simulink model "TST_ActMod_TrqCalc"  (R2016b)
settings: Solver=FixedStepDiscrete  StartTime=0.0  StopTime=0.04  FixedStep=sampleTime  RelTol=1e-3
values from neighbouring files (symbols this model uses):
  testCase = 1    [initTST_ActMod_TrqCalc_001.m]
libraries: simulink x7, UnitTest_Lib x5
settings Model: Creator=caijinkang  LastModifiedBy=caijinkang
settings DebuggingCC: SignalRangeChecking=error

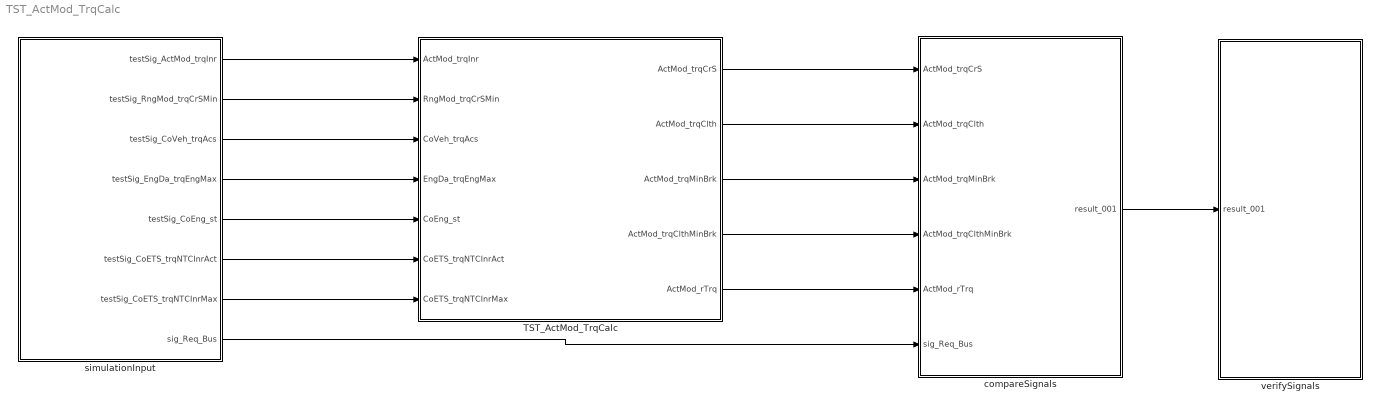
== system TST_ActMod_TrqCalc ==
  TST_ActMod_TrqCalc : Subsystem
  compareSignals : Subsystem
  simulationInput : Subsystem
  verifySignals : Subsystem
  wires:
  simulationInput/1(testSig_ActMod_trqInr) -> TST_ActMod_TrqCalc/1(ActMod_trqInr)
  simulationInput/2(testSig_RngMod_trqCrSMin) -> TST_ActMod_TrqCalc/2(RngMod_trqCrSMin)
  simulationInput/3(testSig_CoVeh_trqAcs) -> TST_ActMod_TrqCalc/3(CoVeh_trqAcs)
  simulationInput/4(testSig_EngDa_trqEngMax) -> TST_ActMod_TrqCalc/4(EngDa_trqEngMax)
  simulationInput/5(testSig_CoEng_st) -> TST_ActMod_TrqCalc/5(CoEng_st)
  simulationInput/6(testSig_CoETS_trqNTCInrAct) -> TST_ActMod_TrqCalc/6(CoETS_trqNTCInrAct)
  simulationInput/7(testSig_CoETS_trqNTCInrMax) -> TST_ActMod_TrqCalc/7(CoETS_trqNTCInrMax)
  TST_ActMod_TrqCalc/1(ActMod_trqCrS) -> compareSignals/1(ActMod_trqCrS)
  TST_ActMod_TrqCalc/2(ActMod_trqClth) -> compareSignals/2(ActMod_trqClth)
  TST_ActMod_TrqCalc/3(ActMod_trqMinBrk) -> compareSignals/3(ActMod_trqMinBrk)
  TST_ActMod_TrqCalc/4(ActMod_trqClthMinBrk) -> compareSignals/4(ActMod_trqClthMinBrk)
  TST_ActMod_TrqCalc/5(ActMod_rTrq) -> compareSignals/5(ActMod_rTrq)
  simulationInput/8(sig_Req_Bus) -> compareSignals/6(sig_Req_Bus)
  compareSignals/1(result_001) -> verifySignals/1(result_001)

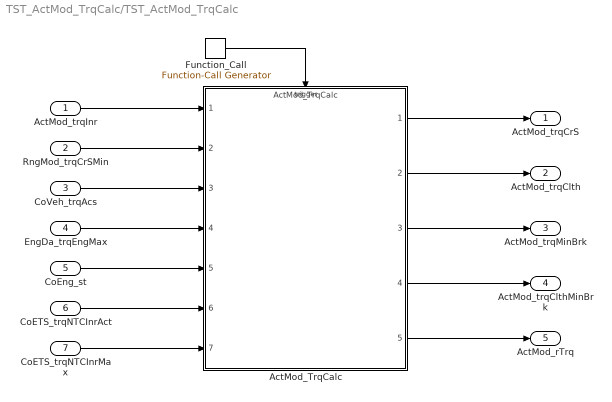
== system TST_ActMod_TrqCalc/TST_ActMod_TrqCalc ==
  ActMod_trqInr : Inport
  RngMod_trqCrSMin : Inport  Port=2
  CoVeh_trqAcs : Inport  Port=3
  EngDa_trqEngMax : Inport  Port=4
  CoEng_st : Inport  Port=5
  CoETS_trqNTCInrAct : Inport  Port=6
  CoETS_trqNTCInrMax : Inport  Port=7
  ActMod_TrqCalc : ModelReference  ModelNameDialog=ActMod_TrqCalc  SimulationMode=Normal  ModelReferenceVersion=1.13  TriggerPortName=function  TriggerPortTriggerType=function-call  TriggerPortStatesWhenEnabling=held
  Function_Call : simulink/Ports & Subsystems/Function-Call Generator  sample_time=sampleTime  numberOfIterations=1
  ActMod_trqCrS : Outport
  ActMod_trqClth : Outport  Port=2
  ActMod_trqMinBrk : Outport  Port=3
  ActMod_trqClthMinBrk : Outport  Port=4
  ActMod_rTrq : Outport  Port=5
  wires:
  Function_Call/1 -> ActMod_TrqCalc/Trigger
  ActMod_trqInr/1 -> ActMod_TrqCalc/1
  RngMod_trqCrSMin/1 -> ActMod_TrqCalc/2
  CoVeh_trqAcs/1 -> ActMod_TrqCalc/3
  EngDa_trqEngMax/1 -> ActMod_TrqCalc/4
  CoEng_st/1 -> ActMod_TrqCalc/5
  CoETS_trqNTCInrAct/1 -> ActMod_TrqCalc/6
  CoETS_trqNTCInrMax/1 -> ActMod_TrqCalc/7
  ActMod_TrqCalc/1 -> ActMod_trqCrS/1
  ActMod_TrqCalc/2 -> ActMod_trqClth/1
  ActMod_TrqCalc/3 -> ActMod_trqMinBrk/1
  ActMod_TrqCalc/4 -> ActMod_trqClthMinBrk/1
  ActMod_TrqCalc/5 -> ActMod_rTrq/1

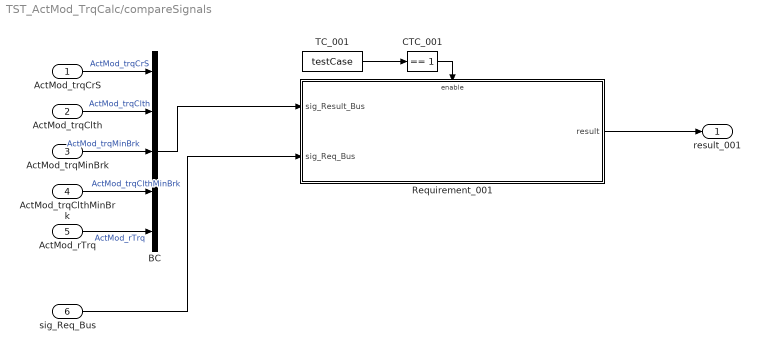
== system TST_ActMod_TrqCalc/compareSignals ==
  ActMod_trqCrS : Inport
  ActMod_trqClth : Inport  Port=2
  ActMod_trqMinBrk : Inport  Port=3
  ActMod_trqClthMinBrk : Inport  Port=4
  ActMod_rTrq : Inport  Port=5
  sig_Req_Bus : Inport  Port=6
  BC : BusCreator  Inputs=5
  CTC_001 : simulink/Logic and Bit Operations/Compare To Constant  relop===  const=1  OutDataTypeStr=boolean
  Requirement_001 : Subsystem
  TC_001 : Constant  Value=testCase
  result_001 : Outport
  wires:
  ActMod_trqCrS/1 -> BC/1  "ActMod_trqCrS"
  ActMod_trqClth/1 -> BC/2  "ActMod_trqClth"
  ActMod_trqMinBrk/1 -> BC/3  "ActMod_trqMinBrk"
  ActMod_trqClthMinBrk/1 -> BC/4  "ActMod_trqClthMinBrk"
  ActMod_rTrq/1 -> BC/5  "ActMod_rTrq"
  TC_001/1 -> CTC_001/1
  CTC_001/1 -> Requirement_001/Enable
  sig_Req_Bus/1 -> Requirement_001/2(sig_Req_Bus)
  BC/1 -> Requirement_001/1(sig_Result_Bus)
  Requirement_001/1(result) -> result_001/1

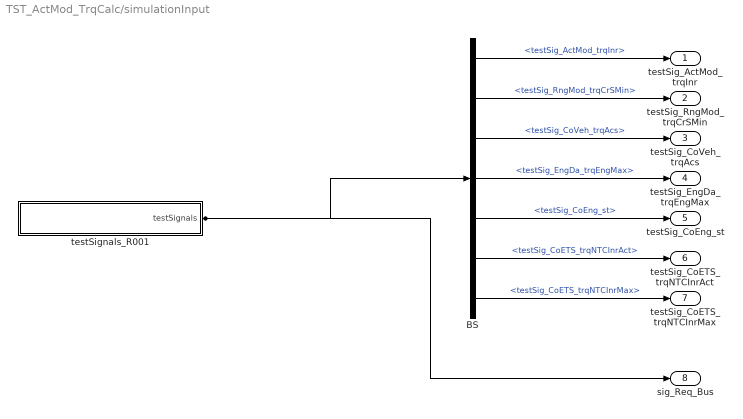
== system TST_ActMod_TrqCalc/simulationInput ==
  BS : BusSelector  OutputSignals=testSig_ActMod_trqInr,testSig_RngMod_trqCrSMin,testSig_CoVeh_trqAcs,testSig_EngDa_trqEngMax,testSig_CoEng_st,testSig_CoETS_trqNTCInrAct,testSig_CoETS_trqNTCInrMax
  testSignals_R001 : Subsystem
  testSig_ActMod_trqInr : Outport
  testSig_RngMod_trqCrSMin : Outport  Port=2
  testSig_CoVeh_trqAcs : Outport  Port=3
  testSig_EngDa_trqEngMax : Outport  Port=4
  testSig_CoEng_st : Outport  Port=5
  testSig_CoETS_trqNTCInrAct : Outport  Port=6
  testSig_CoETS_trqNTCInrMax : Outport  Port=7
  sig_Req_Bus : Outport  Port=8
  wires:
  BS/1 -> testSig_ActMod_trqInr/1  "<testSig_ActMod_trqInr>"
  BS/2 -> testSig_RngMod_trqCrSMin/1  "<testSig_RngMod_trqCrSMin>"
  BS/3 -> testSig_CoVeh_trqAcs/1  "<testSig_CoVeh_trqAcs>"
  BS/4 -> testSig_EngDa_trqEngMax/1  "<testSig_EngDa_trqEngMax>"
  BS/5 -> testSig_CoEng_st/1  "<testSig_CoEng_st>"
  BS/6 -> testSig_CoETS_trqNTCInrAct/1  "<testSig_CoETS_trqNTCInrAct>"
  BS/7 -> testSig_CoETS_trqNTCInrMax/1  "<testSig_CoETS_trqNTCInrMax>"
  testSignals_R001/1(testSignals) -> BS/1, sig_Req_Bus/1

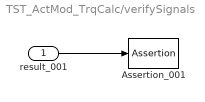
== system TST_ActMod_TrqCalc/verifySignals ==
  result_001 : Inport
  Assertion_001 : Assertion  Enabled=off
  wires:
  result_001/1 -> Assertion_001/1

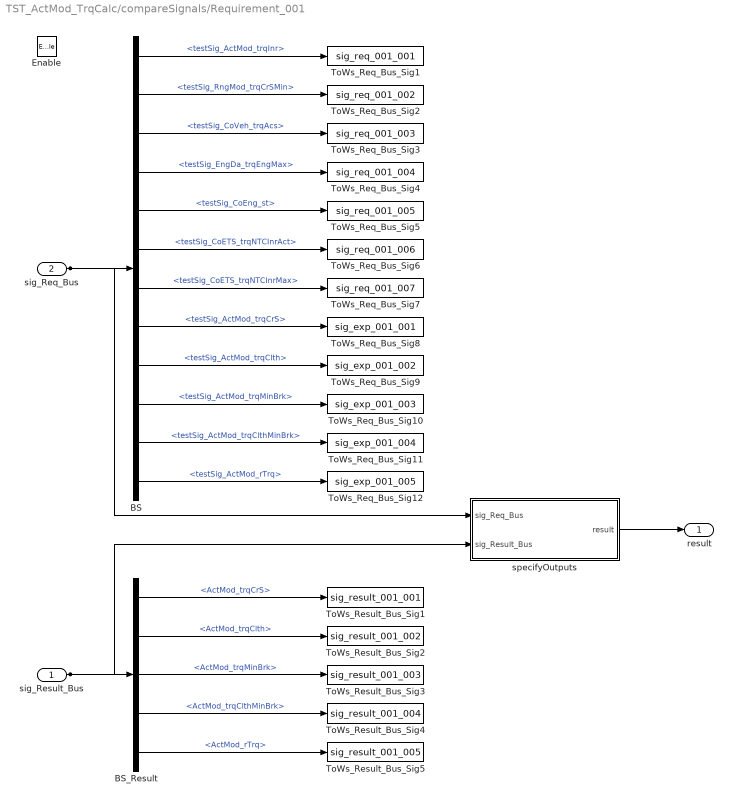
== system TST_ActMod_TrqCalc/compareSignals/Requirement_001 ==
  sig_Result_Bus : Inport
  sig_Req_Bus : Inport  Port=2
  Enable : EnablePort
  BS : BusSelector  OutputSignals=testSig_ActMod_trqInr,testSig_RngMod_trqCrSMin,testSig_CoVeh_trqAcs,testSig_EngDa_trqEngMax,testSig_CoEng_st,testSig_CoETS_trqNTCInrAct,testSig_CoETS_trqNTCInrMax,testSig_ActMod_trqCrS,testSig_ActMod_trqClth,testSig_ActMod_trqMinBrk,testSig_ActMod_trqClthMinBrk,testSig_ActMod_rTrq
  BS_Result : BusSelector  OutputSignals=ActMod_trqCrS,ActMod_trqClth,ActMod_trqMinBrk,ActMod_trqClthMinBrk,ActMod_rTrq
  ToWs_Req_Bus_Sig1 : ToWorkspace  VariableName=sig_req_001_001  SaveFormat=Structure With Time
  ToWs_Req_Bus_Sig10 : ToWorkspace  VariableName=sig_exp_001_003  SaveFormat=Structure With Time
  ToWs_Req_Bus_Sig11 : ToWorkspace  VariableName=sig_exp_001_004  SaveFormat=Structure With Time
  ToWs_Req_Bus_Sig12 : ToWorkspace  VariableName=sig_exp_001_005  SaveFormat=Structure With Time
  ToWs_Req_Bus_Sig2 : ToWorkspace  VariableName=sig_req_001_002  SaveFormat=Structure With Time
  ToWs_Req_Bus_Sig3 : ToWorkspace  VariableName=sig_req_001_003  SaveFormat=Structure With Time
  ToWs_Req_Bus_Sig4 : ToWorkspace  VariableName=sig_req_001_004  SaveFormat=Structure With Time
  ToWs_Req_Bus_Sig5 : ToWorkspace  VariableName=sig_req_001_005  SaveFormat=Structure With Time
  ToWs_Req_Bus_Sig6 : ToWorkspace  VariableName=sig_req_001_006  SaveFormat=Structure With Time
  ToWs_Req_Bus_Sig7 : ToWorkspace  VariableName=sig_req_001_007  SaveFormat=Structure With Time
  ToWs_Req_Bus_Sig8 : ToWorkspace  VariableName=sig_exp_001_001  SaveFormat=Structure With Time
  ToWs_Req_Bus_Sig9 : ToWorkspace  VariableName=sig_exp_001_002  SaveFormat=Structure With Time
  ToWs_Result_Bus_Sig1 : ToWorkspace  VariableName=sig_result_001_001  SaveFormat=Structure With Time
  ToWs_Result_Bus_Sig2 : ToWorkspace  VariableName=sig_result_001_002  SaveFormat=Structure With Time
  ToWs_Result_Bus_Sig3 : ToWorkspace  VariableName=sig_result_001_003  SaveFormat=Structure With Time
  ToWs_Result_Bus_Sig4 : ToWorkspace  VariableName=sig_result_001_004  SaveFormat=Structure With Time
  ToWs_Result_Bus_Sig5 : ToWorkspace  VariableName=sig_result_001_005  SaveFormat=Structure With Time
  specifyOutputs : Subsystem
  result : Outport
  wires:
  sig_Req_Bus/1 -> BS/1, specifyOutputs/1(sig_Req_Bus)
  BS/1 -> ToWs_Req_Bus_Sig1/1  "<testSig_ActMod_trqInr>"
  BS/2 -> ToWs_Req_Bus_Sig2/1  "<testSig_RngMod_trqCrSMin>"
  BS/3 -> ToWs_Req_Bus_Sig3/1  "<testSig_CoVeh_trqAcs>"
  BS/4 -> ToWs_Req_Bus_Sig4/1  "<testSig_EngDa_trqEngMax>"
  BS/5 -> ToWs_Req_Bus_Sig5/1  "<testSig_CoEng_st>"
  BS/6 -> ToWs_Req_Bus_Sig6/1  "<testSig_CoETS_trqNTCInrAct>"
  BS/7 -> ToWs_Req_Bus_Sig7/1  "<testSig_CoETS_trqNTCInrMax>"
  BS/8 -> ToWs_Req_Bus_Sig8/1  "<testSig_ActMod_trqCrS>"
  BS/9 -> ToWs_Req_Bus_Sig9/1  "<testSig_ActMod_trqClth>"
  BS/10 -> ToWs_Req_Bus_Sig10/1  "<testSig_ActMod_trqMinBrk>"
  BS/11 -> ToWs_Req_Bus_Sig11/1  "<testSig_ActMod_trqClthMinBrk>"
  BS/12 -> ToWs_Req_Bus_Sig12/1  "<testSig_ActMod_rTrq>"
  sig_Result_Bus/1 -> BS_Result/1, specifyOutputs/2(sig_Result_Bus)
  BS_Result/1 -> ToWs_Result_Bus_Sig1/1  "<ActMod_trqCrS>"
  BS_Result/2 -> ToWs_Result_Bus_Sig2/1  "<ActMod_trqClth>"
  BS_Result/3 -> ToWs_Result_Bus_Sig3/1  "<ActMod_trqMinBrk>"
  BS_Result/4 -> ToWs_Result_Bus_Sig4/1  "<ActMod_trqClthMinBrk>"
  BS_Result/5 -> ToWs_Result_Bus_Sig5/1  "<ActMod_rTrq>"
  specifyOutputs/1(result) -> result/1

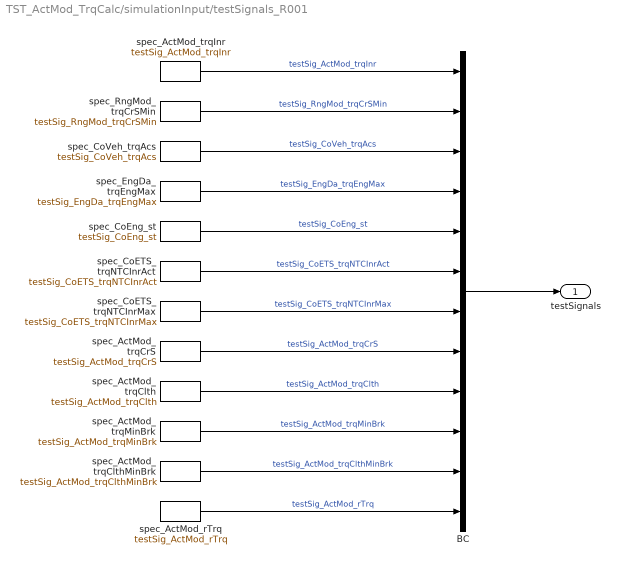
== system TST_ActMod_TrqCalc/simulationInput/testSignals_R001 ==
  BC : BusCreator  Inputs=12
  spec_ActMod_rTrq : FromWorkspace  VariableName=testSig_ActMod_rTrq  Interpolate=off  OutputAfterFinalValue=Holding final value
  spec_ActMod_trqClth : FromWorkspace  VariableName=testSig_ActMod_trqClth  Interpolate=off  OutputAfterFinalValue=Holding final value
  spec_ActMod_trqClthMinBrk : FromWorkspace  VariableName=testSig_ActMod_trqClthMinBrk  Interpolate=off  OutputAfterFinalValue=Holding final value
  spec_ActMod_trqCrS : FromWorkspace  VariableName=testSig_ActMod_trqCrS  Interpolate=off  OutputAfterFinalValue=Holding final value
  spec_ActMod_trqInr : FromWorkspace  VariableName=testSig_ActMod_trqInr  Interpolate=off  OutputAfterFinalValue=Holding final value
  spec_ActMod_trqMinBrk : FromWorkspace  VariableName=testSig_ActMod_trqMinBrk  Interpolate=off  OutputAfterFinalValue=Holding final value
  spec_CoETS_trqNTCInrAct : FromWorkspace  VariableName=testSig_CoETS_trqNTCInrAct  Interpolate=off  OutputAfterFinalValue=Holding final value
  spec_CoETS_trqNTCInrMax : FromWorkspace  VariableName=testSig_CoETS_trqNTCInrMax  Interpolate=off  OutputAfterFinalValue=Holding final value
  spec_CoEng_st : FromWorkspace  VariableName=testSig_CoEng_st  Interpolate=off  OutputAfterFinalValue=Holding final value
  spec_CoVeh_trqAcs : FromWorkspace  VariableName=testSig_CoVeh_trqAcs  Interpolate=off  OutputAfterFinalValue=Holding final value
  spec_EngDa_trqEngMax : FromWorkspace  VariableName=testSig_EngDa_trqEngMax  Interpolate=off  OutputAfterFinalValue=Holding final value
  spec_RngMod_trqCrSMin : FromWorkspace  VariableName=testSig_RngMod_trqCrSMin  Interpolate=off  OutputAfterFinalValue=Holding final value
  testSignals : Outport
  wires:
  BC/1 -> testSignals/1
  spec_ActMod_trqInr/1 -> BC/1  "testSig_ActMod_trqInr"
  spec_RngMod_trqCrSMin/1 -> BC/2  "testSig_RngMod_trqCrSMin"
  spec_CoVeh_trqAcs/1 -> BC/3  "testSig_CoVeh_trqAcs"
  spec_EngDa_trqEngMax/1 -> BC/4  "testSig_EngDa_trqEngMax"
  spec_CoEng_st/1 -> BC/5  "testSig_CoEng_st"
  spec_CoETS_trqNTCInrAct/1 -> BC/6  "testSig_CoETS_trqNTCInrAct"
  spec_CoETS_trqNTCInrMax/1 -> BC/7  "testSig_CoETS_trqNTCInrMax"
  spec_ActMod_trqCrS/1 -> BC/8  "testSig_ActMod_trqCrS"
  spec_ActMod_trqClth/1 -> BC/9  "testSig_ActMod_trqClth"
  spec_ActMod_trqMinBrk/1 -> BC/10  "testSig_ActMod_trqMinBrk"
  spec_ActMod_trqClthMinBrk/1 -> BC/11  "testSig_ActMod_trqClthMinBrk"
  spec_ActMod_rTrq/1 -> BC/12  "testSig_ActMod_rTrq"

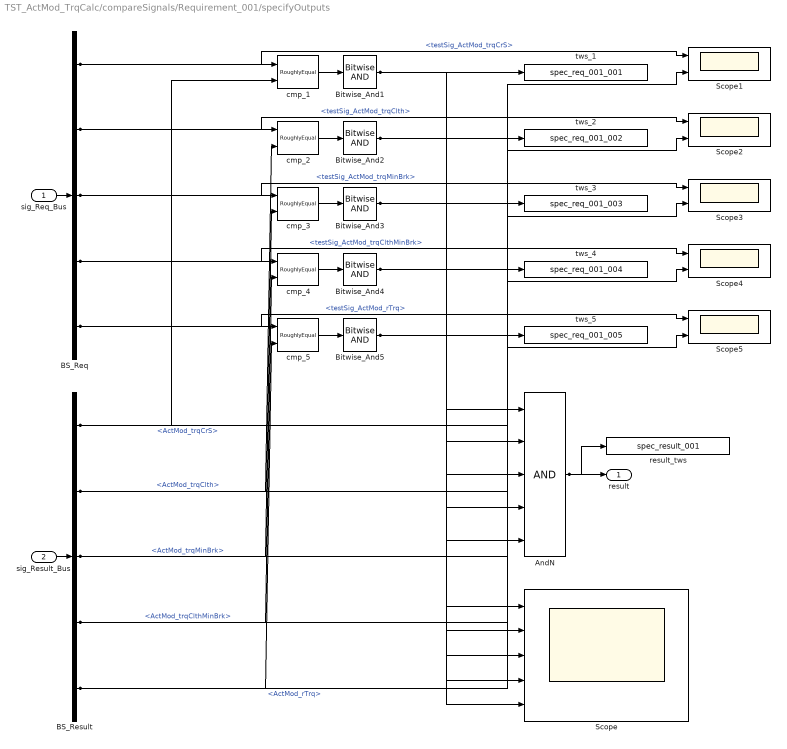
== system TST_ActMod_TrqCalc/compareSignals/Requirement_001/specifyOutputs ==
  sig_Req_Bus : Inport
  sig_Result_Bus : Inport  Port=2
  AndN : Logic  Inputs=5
  BS_Req : BusSelector  OutputSignals=testSig_ActMod_trqCrS,testSig_ActMod_trqClth,testSig_ActMod_trqMinBrk,testSig_ActMod_trqClthMinBrk,testSig_ActMod_rTrq
  BS_Result : BusSelector  OutputSignals=ActMod_trqCrS,ActMod_trqClth,ActMod_trqMinBrk,ActMod_trqClthMinBrk,ActMod_rTrq
  Bitwise_And{1..5} (5 alike) : simulink/Logic and Bit Operations/Bitwise Operator  logicop=AND  UseBitMask=off  BitMask=bin2dec('11011001')  BitMaskRealWorld=Stored Integer
  Scope : Scope  NumInputPorts=5
  Scope{1..5} (5 alike) : Scope  NumInputPorts=2
  cmp_{1..5} (5 alike) : UnitTest_Lib/RoughlyEqual  slope=0.1
  result_tws : ToWorkspace  VariableName=spec_result_001
  tws_1 : ToWorkspace  VariableName=spec_req_001_001
  tws_2 : ToWorkspace  VariableName=spec_req_001_002
  tws_3 : ToWorkspace  VariableName=spec_req_001_003
  tws_4 : ToWorkspace  VariableName=spec_req_001_004
  tws_5 : ToWorkspace  VariableName=spec_req_001_005
  result : Outport
  wires:
  sig_Req_Bus/1 -> BS_Req/1
  sig_Result_Bus/1 -> BS_Result/1
  AndN/1 -> result/1, result_tws/1
  BS_Req/1 -> cmp_1/1, Scope1/1  "<testSig_ActMod_trqCrS>"
  BS_Result/1 -> cmp_1/2, Scope1/2  "<ActMod_trqCrS>"
  cmp_1/1 -> Bitwise_And1/1
  Bitwise_And1/1 -> tws_1/1, AndN/1, Scope/1
  BS_Req/2 -> cmp_2/1, Scope2/1  "<testSig_ActMod_trqClth>"
  BS_Result/2 -> cmp_2/2, Scope2/2  "<ActMod_trqClth>"
  cmp_2/1 -> Bitwise_And2/1
  Bitwise_And2/1 -> tws_2/1, AndN/2, Scope/2
  BS_Req/3 -> cmp_3/1, Scope3/1  "<testSig_ActMod_trqMinBrk>"
  BS_Result/3 -> cmp_3/2, Scope3/2  "<ActMod_trqMinBrk>"
  cmp_3/1 -> Bitwise_And3/1
  Bitwise_And3/1 -> tws_3/1, AndN/3, Scope/3
  BS_Req/4 -> cmp_4/1, Scope4/1  "<testSig_ActMod_trqClthMinBrk>"
  BS_Result/4 -> cmp_4/2, Scope4/2  "<ActMod_trqClthMinBrk>"
  cmp_4/1 -> Bitwise_And4/1
  Bitwise_And4/1 -> tws_4/1, AndN/4, Scope/4
  BS_Req/5 -> cmp_5/1, Scope5/1  "<testSig_ActMod_rTrq>"
  BS_Result/5 -> cmp_5/2, Scope5/2  "<ActMod_rTrq>"
  cmp_5/1 -> Bitwise_And5/1
  Bitwise_And5/1 -> tws_5/1, AndN/5, Scope/5
